simulink model "Multibody_Street_Drone"  (R2019b)
settings: Solver=FixedStepAuto  StartTime=0.0  StopTime=20  FixedStep=0.0075  MaxStep=1e-1  MinStep=1e-7  RelTol=1e-3  AbsTol=1e-6
values from neighbouring files (symbols this model uses):
  Rear_brake = [0 1.82218650851 3.8277518469 5.98774429698 7.94202318038 9.84492098434 11.9533431061 13.8561462856 16.0160441112 18.021704074 19.9760775819 21.9303564653 ... (72 elements, 36x2)]    [Rear_brake.mat]
  TPS_0 = [469.425704648 608.284708657 814.443475346 1022.3060335 1213.13067704 1420.75786613 1608.14616582 1820.50021131 2024.31741075 2213.1951296 2423.41496358 2611.22557668 ... (88 elements, 44x2)]    [TPS_0.mat]
undefined symbols (not defined in the file or in its folder): Front_brake, sigbuilder_block, X, Y, Z
libraries: sm_lib x290, nesl_utility x136, simulink x2
(part 12 of 12)

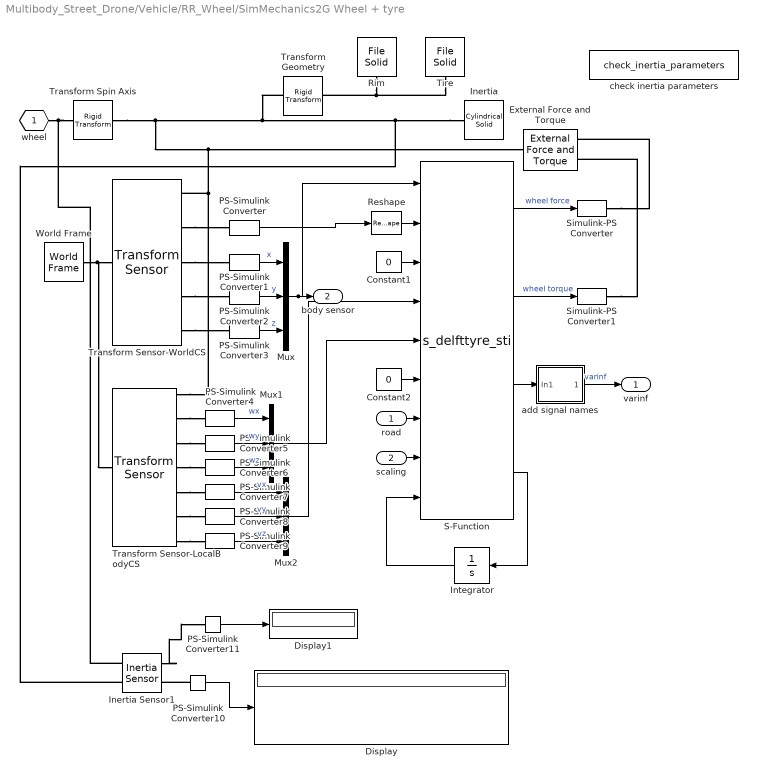
== system Multibody_Street_Drone/Vehicle/RR_Wheel/SimMechanics2G Wheel + tyre ==
  road : Inport
  scaling : Inport  Port=2
  Constant1 : Constant  Value=0
  Constant2 : Constant  Value=0
  Display : Display
  Display1 : Display
  External Force and Torque : sm_lib/Forces and Torques/External Force and Torque  ForceResolutionFrame=AttachedFrame  EnableForceX=off  EnableForceY=off  EnableForceZ=off  EnableForce=on  TorqueResolutionFrame=AttachedFrame  EnableTorqueX=off  EnableTorqueY=off  EnableTorqueZ=off  EnableTorque=on
  Inertia : sm_lib/Body Elements/Cylindrical Solid  GraphicAmbientColor=[0.15 0.15 0.15 1.0]  BasedOnType=Density  CenterOfMass=[0 0 0]  CenterOfMassUnits=m  GraphicDiffuseColor=[0.2 0.8 1.0]  CylinderLength=0.001  CylinderLengthUnits=m  CylinderRadius=0.001  CylinderRadiusUnits=m  Density=1000  DensityUnits=kg/(m^3)  DoExposeReferenceFrame=on  GraphicEmissiveColor=[0.0 0.0 0.0 1.0]  ExportEntireGeometry=off  SerializedFrames=<Frames/>  MarkerShape=Sphere  MarkerSize=10  GraphicType=FromGeometry  InertiaType=Custom  Mass=mass  MassUnits=kg  MomentsOfInertia=[Imat(1,1) Imat(2,2) Imat(3,3)]  MomentsOfInertiaUnits=kg*m^2  GraphicOpacity=1.0  ProductsOfInertia=[0 0 0]  ProductsOfInertiaUnits=kg*m^2  GraphicShininess=75  GraphicSpecularColor=[0.5 0.5 0.5 1.0]  GraphicVisPropType=SimpleVisualProperties
  Inertia Sensor1 : sm_lib/Body Elements/Inertia Sensor  SensorExtent=BodyGroup  SpanWeldJoints=off  ExcludeGroundedBodies=off  MeasurementFrame=Custom  SenseMass=on  SenseCenterOfMass=off  SenseInertiaMatrix=on  SenseCenteredInertiaMatrix=off  SensePrincipalInertiaMatrix=off  SenseRotationMatrix=off  GraphicType=PrincipalInertiaFrame  PrincipalInertiaFrameSize=20  GraphicVisPropType=SimpleVisualProperties  GraphicDiffuseColor=[0.5 0.5 0.5]  GraphicSpecularColor=[0.5 0.5 0.5 1.0]  GraphicAmbientColor=[0.15 0.15 0.15 1.0]  GraphicEmissiveColor=[0.0 0.0 0.0 1.0]  GraphicShininess=75  GraphicOpacity=1.0
      settings: SourceProductBaseCode=MS
  Integrator : Integrator  InitialCondition=zeros(1,40)
  Mux : Mux  Inputs=3
  Mux1 : Mux  Inputs=3
  Mux2 : Mux  Inputs=3
  PS-Simulink Converter{,1..9} (10 alike) : nesl_utility/PS-Simulink Converter  PhysicalDomain=network_engine_domain  SubClassName=ps_output  LeftPortType=input  RightPortType=output  PseudoPeriodic=off  Frequencies=[]  Unit=1  AffineConversion=off
  PS-Simulink Converter10 : nesl_utility/PS-Simulink Converter  PhysicalDomain=network_engine_domain  SubClassName=ps_output  LeftPortType=input  RightPortType=output  PseudoPeriodic=off  Frequencies=[]  Unit=inherit  AffineConversion=off
  PS-Simulink Converter11 : nesl_utility/PS-Simulink Converter  PhysicalDomain=network_engine_domain  SubClassName=ps_output  LeftPortType=input  RightPortType=output  PseudoPeriodic=off  Frequencies=[]  Unit=inherit  AffineConversion=off
  Reshape : Reshape
  Rim : sm_lib/Body Elements/File Solid  ExtGeomFileName=D:\Project\PATH PLANNER STREET DRONE - 618341\CAD geometry\Rim_Back.stl  UnitType=Custom  ExtGeomFileUnits=mm  StepReaderType=HEX  ExportEntireGeometry=off  InertiaType=Custom  Mass=0  MassUnits=kg  CenterOfMass=[0 0 0]  CenterOfMassUnits=m  MomentsOfInertia=[0 0 0]  MomentsOfInertiaUnits=kg*m^2  ProductsOfInertia=[0 0 0]  ProductsOfInertiaUnits=kg*m^2  BasedOnType=Density  Density=1000  DensityUnits=kg/(m^3)  DoExposeReferenceFrame=on  SerializedFrames=<Frames/>  GraphicType=FromGeometry  MarkerShape=Sphere  MarkerSize=10  MarkerSizeUnits=m  GraphicVisPropType=SimpleVisualProperties  GraphicDiffuseColor=[0.8 0.8 0.8]  GraphicSpecularColor=[0.5 0.5 0.5 1.0]  GraphicAmbientColor=[0.15 0.15 0.15 1.0]  GraphicEmissiveColor=[0.0 0.0 0.0 1.0]  GraphicShininess=75  GraphicOpacity=1.0
  S-Function : S-Function  FunctionName=s_delfttyre_sti  Parameters=iswtch idtyre idroad tpfname_dummy rdfname typarr  SFunctionDeploymentMode=off  EnableBusSupport=off
  Simulink-PS Converter : nesl_utility/Simulink-PS Converter  PhysicalDomain=network_engine_domain  SubClassName=ps_input  LeftPortType=input  RightPortType=output  PseudoPeriodic=off  Frequencies=[]  NoiseDistribution=none  NoiseParameters=[]  Unit=1  AffineConversion=off  FilteringAndDerivatives=zero  SimscapeFilterOrder=1  InputFilterTimeConstant=0.001  UdotUserProvided=1
  Simulink-PS Converter1 : nesl_utility/Simulink-PS Converter  PhysicalDomain=network_engine_domain  SubClassName=ps_input  LeftPortType=input  RightPortType=output  PseudoPeriodic=off  Frequencies=[]  NoiseDistribution=none  NoiseParameters=[]  Unit=1  AffineConversion=off  FilteringAndDerivatives=zero  SimscapeFilterOrder=1  InputFilterTimeConstant=0.001  UdotUserProvided=1
  Tire : sm_lib/Body Elements/File Solid  ExtGeomFileName=D:\Project\PATH PLANNER STREET DRONE - 618341\CAD geometry\Tire_Back.stl  UnitType=Custom  ExtGeomFileUnits=mm  StepReaderType=HEX  ExportEntireGeometry=off  InertiaType=Custom  Mass=0  MassUnits=kg  CenterOfMass=[0 0 0]  CenterOfMassUnits=m  MomentsOfInertia=[0 0 0]  MomentsOfInertiaUnits=kg*m^2  ProductsOfInertia=[0 0 0]  ProductsOfInertiaUnits=kg*m^2  BasedOnType=Density  Density=1000  DensityUnits=kg/(m^3)  DoExposeReferenceFrame=on  SerializedFrames=<Frames/>  GraphicType=FromGeometry  MarkerShape=Sphere  MarkerSize=10  MarkerSizeUnits=m  GraphicVisPropType=SimpleVisualProperties  GraphicDiffuseColor=[0.5 0.5 0.5]  GraphicSpecularColor=[0.5 0.5 0.5 1.0]  GraphicAmbientColor=[0.15 0.15 0.15 1.0]  GraphicEmissiveColor=[0.0 0.0 0.0 1.0]  GraphicShininess=75  GraphicOpacity=1.0
  Transform Geometry : sm_lib/Frames and Transforms/Rigid Transform  TranslationMethod=StandardAxis  TranslationStandardOffset=(1-2*fliplr)*0.125  TranslationLengthUnit=m  TranslationStandardAxis=+Y  TranslationCartesianOffset=[0 0 0]  TranslationROffset=0  TranslationROffsetUnits=m  TranslationZOffset=0  TranslationZOffsetUnits=m  TranslationThetaOffset=0  TranslationThetaOffsetUnits=deg  RotationMethod=StandardAxis  RotationAngleUnits=deg  RotationStandardAxis=+X  RotationAngle=fliplr*180-90  RotationArbitraryAxis=[0 0 1]  FollAlignAxisA=+X  BaseAlignAxisA=+Y  FollAlignAxisB=+Y  BaseAlignAxisB=+Z  RotationSequenceAxes=FollowerAxes  RotationSequence=XYX  RotationSequenceAngles=[0 0 0]  RotationSequenceAnglesUnits=deg  RotationMatrix=[1 0 0; 0 1 0; 0 0 1]
  Transform Sensor-LocalBodyCS : sm_lib/Frames and Transforms/Transform Sensor  MeasurementFrame=NonRotatingFollower  SenseAngle=off  SenseAxis=off  SenseAngle1=off  SenseAngle2=off  SenseAngle3=off  SenseQ=off  SenseR=off  SenseOmegaX=on  SenseOmegaY=on  SenseOmegaZ=on  SenseOmega1=off  SenseOmega2=off  SenseOmega3=off  SenseQDot=off  SenseRDot=off  SenseAlphaX=off  SenseAlphaY=off  SenseAlphaZ=off  SenseAlpha1=off  SenseAlpha2=off  SenseAlpha3=off  SenseQDDot=off  SenseRDDot=off  SenseX=off  SenseY=off  SenseZ=off  SenseRad=off  SenseAzim=off  SenseDist=off  SenseInc=off  SenseXDot=on  SenseYDot=on  SenseZDot=on  SenseRadDot=off  SenseAzimDot=off  SenseDistDot=off  SenseIncDot=off  SenseXDDot=off  SenseYDDot=off  SenseZDDot=off  SenseRadDDot=off  SenseAzimDDot=off  SenseDistDDot=off  SenseIncDDot=off
  Transform Sensor-WorldCS : sm_lib/Frames and Transforms/Transform Sensor  MeasurementFrame=World  SenseAngle=off  SenseAxis=off  SenseAngle1=off  SenseAngle2=off  SenseAngle3=off  SenseQ=off  SenseR=on  SenseOmegaX=off  SenseOmegaY=off  SenseOmegaZ=off  SenseOmega1=off  SenseOmega2=off  SenseOmega3=off  SenseQDot=off  SenseRDot=off  SenseAlphaX=off  SenseAlphaY=off  SenseAlphaZ=off  SenseAlpha1=off  SenseAlpha2=off  SenseAlpha3=off  SenseQDDot=off  SenseRDDot=off  SenseX=on  SenseY=on  SenseZ=on  SenseRad=off  SenseAzim=off  SenseDist=off  SenseInc=off  SenseXDot=off  SenseYDot=off  SenseZDot=off  SenseRadDot=off  SenseAzimDot=off  SenseDistDot=off  SenseIncDot=off  SenseXDDot=off  SenseYDDot=off  SenseZDDot=off  SenseRadDDot=off  SenseAzimDDot=off  SenseDistDDot=off  SenseIncDDot=off
  Transform Spin Axis : sm_lib/Frames and Transforms/Rigid Transform  TranslationMethod=None  TranslationStandardOffset=0  TranslationLengthUnit=m  TranslationStandardAxis=+Z  TranslationCartesianOffset=[0 0 0]  TranslationROffset=0  TranslationROffsetUnits=m  TranslationZOffset=0  TranslationZOffsetUnits=m  TranslationThetaOffset=0  TranslationThetaOffsetUnits=deg  RotationMethod=StandardAxis  RotationAngleUnits=deg  RotationStandardAxis=-X  RotationAngle=90  RotationArbitraryAxis=[0 0 1]  FollAlignAxisA=+X  BaseAlignAxisA=+Y  FollAlignAxisB=+Y  BaseAlignAxisB=+Z  RotationSequenceAxes=FollowerAxes  RotationSequence=XYX  RotationSequenceAngles=[0 0 0]  RotationSequenceAnglesUnits=deg  RotationMatrix=[1 0 0; 0 1 0; 0 0 1]
  World Frame : sm_lib/Frames and Transforms/World Frame
  add signal names : Subsystem
  check inertia parameters : M-S-Function  Priority=1  FunctionName=check_inertia_parameters  Parameters=tpfname1, rdfname1, typarr1  mask{tpfname1=tpfname_dummy, rdfname1=rdfname, typarr1=typarr}
      mask prompts: tpfname1 "Tyre Property File"; rdfname1 "Road Data File"; typarr1 "typarr"
      mask help: Checks Inertia parameters as calculated in mask
  wheel : PMIOPort  Side=Left
  varinf : Outport
  body sensor : Outport  Port=2
  wires:
  Reshape/1 -> S-Function/2
  S-Function/1 -> Simulink-PS Converter/1  "wheel force"
  S-Function/2 -> Simulink-PS Converter1/1  "wheel torque"
  Mux/1 -> S-Function/1, body sensor/1
  PS-Simulink Converter9/1 -> Mux2/3  "vz"
  PS-Simulink Converter8/1 -> Mux2/2  "vy"
  PS-Simulink Converter7/1 -> Mux2/1  "vx"
  PS-Simulink Converter6/1 -> Mux1/3  "wz"
  PS-Simulink Converter5/1 -> Mux1/2  "wy"
  PS-Simulink Converter4/1 -> Mux1/1  "wx"
  PS-Simulink Converter3/1 -> Mux/3  "z"
  PS-Simulink Converter2/1 -> Mux/2  "y"
  PS-Simulink Converter1/1 -> Mux/1  "x"
  Constant1/1 -> S-Function/3
  Integrator/1 -> S-Function/9
  scaling/1 -> S-Function/8
  road/1 -> S-Function/7
  add signal names/1(Out1) -> varinf/1  "varinf"
  S-Function/3 -> add signal names/1(In1)
  S-Function/4 -> Integrator/1
  PS-Simulink Converter/1 -> Reshape/1
  Mux1/1 -> S-Function/5
  Mux2/1 -> S-Function/4
  Constant2/1 -> S-Function/6
  PS-Simulink Converter10/1 -> Display/1
  PS-Simulink Converter11/1 -> Display1/1
  connections:
  Transform Sensor-WorldCS/LConn1 -- World Frame/RConn1 -- Transform Sensor-LocalBodyCS/LConn1
  Inertia/RConn1 -- Transform Spin Axis/LConn1 -- Transform Sensor-WorldCS/RConn1 -- Transform Sensor-LocalBodyCS/RConn1 -- External Force and Torque/RConn1 -- Transform Geometry/LConn1 -- Inertia Sensor1/LConn2
  Transform Geometry/RConn1 -- Rim/RConn1 -- Tire/RConn1
  Transform Sensor-LocalBodyCS/RConn7 -- PS-Simulink Converter9/LConn1
  Transform Sensor-LocalBodyCS/RConn6 -- PS-Simulink Converter8/LConn1
  Transform Sensor-LocalBodyCS/RConn5 -- PS-Simulink Converter7/LConn1
  Transform Sensor-LocalBodyCS/RConn4 -- PS-Simulink Converter6/LConn1
  Transform Sensor-LocalBodyCS/RConn3 -- PS-Simulink Converter5/LConn1
  Transform Sensor-LocalBodyCS/RConn2 -- PS-Simulink Converter4/LConn1
  Transform Sensor-WorldCS/RConn5 -- PS-Simulink Converter3/LConn1
  Transform Sensor-WorldCS/RConn4 -- PS-Simulink Converter2/LConn1
  Transform Sensor-WorldCS/RConn3 -- PS-Simulink Converter1/LConn1
  Transform Sensor-WorldCS/RConn2 -- PS-Simulink Converter/LConn1
  Simulink-PS Converter/RConn1 -- External Force and Torque/LConn1
  Simulink-PS Converter1/RConn1 -- External Force and Torque/LConn2
  Transform Spin Axis/RConn1 -- wheel/RConn1 -- Inertia Sensor1/LConn1
  PS-Simulink Converter10/LConn1 -- Inertia Sensor1/RConn2
  Inertia Sensor1/RConn1 -- PS-Simulink Converter11/LConn1

== system Multibody_Street_Drone/Results/Fx/Calculated/Torque_inertia ==
  RL : Subsystem
  RR : Subsystem

== system Multibody_Street_Drone/Results/Fx/Calculated/Whole_vehicle ==
  Product : Product
  To Workspace3 : ToWorkspace  VariableName=Calc_Fx_vehicle  SampleTime=-1
  wires:
  [Act_Ax] -> Product/1
  Product/1 -> To Workspace3/1
  [mass] -> Product/2

== system Multibody_Street_Drone/Vehicle/FL_Wheel/SimMechanics2G Wheel + tyre/add signal names ==
  In1 : Inport
  Added for future extension : Terminator
  Bus Creator : BusCreator  Inputs=40
  Demux1 : Demux  Outputs=[ones(1,40) -1]
  Out1 : Outport
  wires:
  Demux1/41 -> Added for future extension/1
  Demux1/40 -> Bus Creator/40  "eff_plane_banking"
  Demux1/39 -> Bus Creator/39  "eff_plane_curvature"
  Demux1/38 -> Bus Creator/38  "eff_plane_angle"
  Demux1/37 -> Bus Creator/37  "eff_plane_height"
  Demux1/36 -> Bus Creator/36  "nz"
  Demux1/35 -> Bus Creator/35  "ny"
  Demux1/34 -> Bus Creator/34  "nx"
  Demux1/33 -> Bus Creator/33  "zcp"
  Demux1/32 -> Bus Creator/32  "ycp"
  Demux1/31 -> Bus Creator/31  "xcp"
  Demux1/30 -> Bus Creator/30  "_e30"
  Demux1/29 -> Bus Creator/29  "_e29"
  Demux1/28 -> Bus Creator/28  "travelled_distance"
  Demux1/27 -> Bus Creator/27  "_e27"
  Demux1/26 -> Bus Creator/26  "_e26"
  Demux1/25 -> Bus Creator/25  "_e25"
  Demux1/24 -> Bus Creator/24  "psidot"
  Demux1/23 -> Bus Creator/23  "Vz"
  Demux1/22 -> Bus Creator/22  "Vsy"
  Demux1/21 -> Bus Creator/21  "Vsx"
  Demux1/20 -> Bus Creator/20  "relaxation_length_y"
  Demux1/19 -> Bus Creator/19  "relaxation_length_x"
  Demux1/18 -> Bus Creator/18  "mu_y"
  Demux1/17 -> Bus Creator/17  "mu_x"
  Demux1/16 -> Bus Creator/16  "pneumatic_trail"
  Demux1/15 -> Bus Creator/15  "contact_length"
  Demux1/14 -> Bus Creator/14  "vertical_deflection"
  Demux1/13 -> Bus Creator/13  "effective_rolling_radius"
  Demux1/12 -> Bus Creator/12  "_e12"
  Demux1/11 -> Bus Creator/11  "Vx"
  Demux1/10 -> Bus Creator/10  "turn_slip"
  Demux1/9 -> Bus Creator/9  "inclination_angle"
  Demux1/8 -> Bus Creator/8  "side_slip_angle"
  Demux1/7 -> Bus Creator/7  "longitudinal_slip"
  Demux1/6 -> Bus Creator/6  "Mz"
  Demux1/5 -> Bus Creator/5  "My"
  Demux1/4 -> Bus Creator/4  "Mx"
  Demux1/3 -> Bus Creator/3  "Fz"
  Demux1/2 -> Bus Creator/2  "Fy"
  Demux1/1 -> Bus Creator/1  "Fx"
  Bus Creator/1 -> Out1/1  "varinf"
  In1/1 -> Demux1/1

== system Multibody_Street_Drone/Vehicle/FR_Wheel/SimMechanics2G Wheel + tyre/add signal names ==
  In1 : Inport
  Added for future extension : Terminator
  Bus Creator : BusCreator  Inputs=40
  Demux1 : Demux  Outputs=[ones(1,40) -1]
  Out1 : Outport
  wires:
  In1/1 -> Demux1/1
  Bus Creator/1 -> Out1/1  "varinf"
  Demux1/1 -> Bus Creator/1  "Fx"
  Demux1/2 -> Bus Creator/2  "Fy"
  Demux1/3 -> Bus Creator/3  "Fz"
  Demux1/4 -> Bus Creator/4  "Mx"
  Demux1/5 -> Bus Creator/5  "My"
  Demux1/6 -> Bus Creator/6  "Mz"
  Demux1/7 -> Bus Creator/7  "longitudinal_slip"
  Demux1/8 -> Bus Creator/8  "side_slip_angle"
  Demux1/9 -> Bus Creator/9  "inclination_angle"
  Demux1/10 -> Bus Creator/10  "turn_slip"
  Demux1/11 -> Bus Creator/11  "Vx"
  Demux1/12 -> Bus Creator/12  "_e12"
  Demux1/13 -> Bus Creator/13  "effective_rolling_radius"
  Demux1/14 -> Bus Creator/14  "vertical_deflection"
  Demux1/15 -> Bus Creator/15  "contact_length"
  Demux1/16 -> Bus Creator/16  "pneumatic_trail"
  Demux1/17 -> Bus Creator/17  "mu_x"
  Demux1/18 -> Bus Creator/18  "mu_y"
  Demux1/19 -> Bus Creator/19  "relaxation_length_x"
  Demux1/20 -> Bus Creator/20  "relaxation_length_y"
  Demux1/21 -> Bus Creator/21  "Vsx"
  Demux1/22 -> Bus Creator/22  "Vsy"
  Demux1/23 -> Bus Creator/23  "Vz"
  Demux1/24 -> Bus Creator/24  "psidot"
  Demux1/25 -> Bus Creator/25  "_e25"
  Demux1/26 -> Bus Creator/26  "_e26"
  Demux1/27 -> Bus Creator/27  "_e27"
  Demux1/28 -> Bus Creator/28  "travelled_distance"
  Demux1/29 -> Bus Creator/29  "_e29"
  Demux1/30 -> Bus Creator/30  "_e30"
  Demux1/31 -> Bus Creator/31  "xcp"
  Demux1/32 -> Bus Creator/32  "ycp"
  Demux1/33 -> Bus Creator/33  "zcp"
  Demux1/34 -> Bus Creator/34  "nx"
  Demux1/35 -> Bus Creator/35  "ny"
  Demux1/36 -> Bus Creator/36  "nz"
  Demux1/37 -> Bus Creator/37  "eff_plane_height"
  Demux1/38 -> Bus Creator/38  "eff_plane_angle"
  Demux1/39 -> Bus Creator/39  "eff_plane_curvature"
  Demux1/40 -> Bus Creator/40  "eff_plane_banking"
  Demux1/41 -> Added for future extension/1

== system Multibody_Street_Drone/Vehicle/RL_Wheel/SimMechanics2G Wheel + tyre/add signal names ==
  In1 : Inport
  Added for future extension : Terminator
  Bus Creator : BusCreator  Inputs=40
  Demux1 : Demux  Outputs=[ones(1,40) -1]
  Out1 : Outport
  wires:
  In1/1 -> Demux1/1
  Bus Creator/1 -> Out1/1  "varinf"
  Demux1/1 -> Bus Creator/1  "Fx"
  Demux1/2 -> Bus Creator/2  "Fy"
  Demux1/3 -> Bus Creator/3  "Fz"
  Demux1/4 -> Bus Creator/4  "Mx"
  Demux1/5 -> Bus Creator/5  "My"
  Demux1/6 -> Bus Creator/6  "Mz"
  Demux1/7 -> Bus Creator/7  "longitudinal_slip"
  Demux1/8 -> Bus Creator/8  "side_slip_angle"
  Demux1/9 -> Bus Creator/9  "inclination_angle"
  Demux1/10 -> Bus Creator/10  "turn_slip"
  Demux1/11 -> Bus Creator/11  "Vx"
  Demux1/12 -> Bus Creator/12  "_e12"
  Demux1/13 -> Bus Creator/13  "effective_rolling_radius"
  Demux1/14 -> Bus Creator/14  "vertical_deflection"
  Demux1/15 -> Bus Creator/15  "contact_length"
  Demux1/16 -> Bus Creator/16  "pneumatic_trail"
  Demux1/17 -> Bus Creator/17  "mu_x"
  Demux1/18 -> Bus Creator/18  "mu_y"
  Demux1/19 -> Bus Creator/19  "relaxation_length_x"
  Demux1/20 -> Bus Creator/20  "relaxation_length_y"
  Demux1/21 -> Bus Creator/21  "Vsx"
  Demux1/22 -> Bus Creator/22  "Vsy"
  Demux1/23 -> Bus Creator/23  "Vz"
  Demux1/24 -> Bus Creator/24  "psidot"
  Demux1/25 -> Bus Creator/25  "_e25"
  Demux1/26 -> Bus Creator/26  "_e26"
  Demux1/27 -> Bus Creator/27  "_e27"
  Demux1/28 -> Bus Creator/28  "travelled_distance"
  Demux1/29 -> Bus Creator/29  "_e29"
  Demux1/30 -> Bus Creator/30  "_e30"
  Demux1/31 -> Bus Creator/31  "xcp"
  Demux1/32 -> Bus Creator/32  "ycp"
  Demux1/33 -> Bus Creator/33  "zcp"
  Demux1/34 -> Bus Creator/34  "nx"
  Demux1/35 -> Bus Creator/35  "ny"
  Demux1/36 -> Bus Creator/36  "nz"
  Demux1/37 -> Bus Creator/37  "eff_plane_height"
  Demux1/38 -> Bus Creator/38  "eff_plane_angle"
  Demux1/39 -> Bus Creator/39  "eff_plane_curvature"
  Demux1/40 -> Bus Creator/40  "eff_plane_banking"
  Demux1/41 -> Added for future extension/1

== system Multibody_Street_Drone/Vehicle/RR_Wheel/SimMechanics2G Wheel + tyre/add signal names ==
  In1 : Inport
  Added for future extension : Terminator
  Bus Creator : BusCreator  Inputs=40
  Demux1 : Demux  Outputs=[ones(1,40) -1]
  Out1 : Outport
  wires:
  Demux1/41 -> Added for future extension/1
  Demux1/40 -> Bus Creator/40  "eff_plane_banking"
  Demux1/39 -> Bus Creator/39  "eff_plane_curvature"
  Demux1/38 -> Bus Creator/38  "eff_plane_angle"
  Demux1/37 -> Bus Creator/37  "eff_plane_height"
  Demux1/36 -> Bus Creator/36  "nz"
  Demux1/35 -> Bus Creator/35  "ny"
  Demux1/34 -> Bus Creator/34  "nx"
  Demux1/33 -> Bus Creator/33  "zcp"
  Demux1/32 -> Bus Creator/32  "ycp"
  Demux1/31 -> Bus Creator/31  "xcp"
  Demux1/30 -> Bus Creator/30  "_e30"
  Demux1/29 -> Bus Creator/29  "_e29"
  Demux1/28 -> Bus Creator/28  "travelled_distance"
  Demux1/27 -> Bus Creator/27  "_e27"
  Demux1/26 -> Bus Creator/26  "_e26"
  Demux1/25 -> Bus Creator/25  "_e25"
  Demux1/24 -> Bus Creator/24  "psidot"
  Demux1/23 -> Bus Creator/23  "Vz"
  Demux1/22 -> Bus Creator/22  "Vsy"
  Demux1/21 -> Bus Creator/21  "Vsx"
  Demux1/20 -> Bus Creator/20  "relaxation_length_y"
  Demux1/19 -> Bus Creator/19  "relaxation_length_x"
  Demux1/18 -> Bus Creator/18  "mu_y"
  Demux1/17 -> Bus Creator/17  "mu_x"
  Demux1/16 -> Bus Creator/16  "pneumatic_trail"
  Demux1/15 -> Bus Creator/15  "contact_length"
  Demux1/14 -> Bus Creator/14  "vertical_deflection"
  Demux1/13 -> Bus Creator/13  "effective_rolling_radius"
  Demux1/12 -> Bus Creator/12  "_e12"
  Demux1/11 -> Bus Creator/11  "Vx"
  Demux1/10 -> Bus Creator/10  "turn_slip"
  Demux1/9 -> Bus Creator/9  "inclination_angle"
  Demux1/8 -> Bus Creator/8  "side_slip_angle"
  Demux1/7 -> Bus Creator/7  "longitudinal_slip"
  Demux1/6 -> Bus Creator/6  "Mz"
  Demux1/5 -> Bus Creator/5  "My"
  Demux1/4 -> Bus Creator/4  "Mx"
  Demux1/3 -> Bus Creator/3  "Fz"
  Demux1/2 -> Bus Creator/2  "Fy"
  Demux1/1 -> Bus Creator/1  "Fx"
  Bus Creator/1 -> Out1/1  "varinf"
  In1/1 -> Demux1/1

== system Multibody_Street_Drone/Results/Fx/Calculated/Torque_inertia/RL ==
  Add : Sum
  Add1 : Sum  Inputs=+-
  Divide2 : Product  Inputs=*/
  Divide3 : Product  Inputs=*/
  Ie : Constant  Value=0.0226
  Iw : Constant  Value=0.4665
  Product2 : Product
  Product3 : Product
  To Workspace1 : ToWorkspace  VariableName=calc_Fx_RL  SampleTime=-1
  tag scope: Iner_loss_L=global
  wires:
  [RL_Re] -> Product3/2
  Divide2/1 -> Add1/1
  Product2/1 -> Divide3/1
  [Act_Ax] -> Product2/2
  [RL_Re] -> Product3/1
  Iw/1 -> Add/2
  [RL_Re] -> Divide2/2
  [Me_Pt] -> Divide2/1
  Ie/1 -> Add/1
  Product3/1 -> Divide3/2
  Divide3/1 -> [Iner_loss_L], Add1/2
  Add1/1 -> To Workspace1/1
  Add/1 -> Product2/1

== system Multibody_Street_Drone/Results/Fx/Calculated/Torque_inertia/RR ==
  Add2 : Sum
  Add3 : Sum  Inputs=+-
  Divide1 : Product  Inputs=*/
  Divide4 : Product  Inputs=*/
  Ie_R : Constant  Value=0.0226
  Iw_R : Constant  Value=0.4665
  Product1 : Product
  Product4 : Product
  To Workspace2 : ToWorkspace  VariableName=calc_Fx_RR  SampleTime=-1
  tag scope: Iner_loss_R=global
  wires:
  Product4/1 -> Divide4/2
  Divide4/1 -> [Iner_loss_R], Add3/2
  [RR_Re] -> Product4/2
  Divide1/1 -> Add3/1
  Add3/1 -> To Workspace2/1
  [RR_Re] -> Product4/1
  Ie_R/1 -> Add2/1
  [Act_Ax] -> Product1/2
  [RR_Re] -> Divide1/2
  Product1/1 -> Divide4/1
  Iw_R/1 -> Add2/2
  [Me_Pt] -> Divide1/1
  Add2/1 -> Product1/1
